simulink model "vehicle_simulation_wCOMM"  (R2018b)
settings: Solver=ode4  StartTime=0.0  StopTime=2  FixedStep=0.001  RelTol=1e-3
undefined symbols (not defined in the file): HDBK, MIL, serial
libraries: powerlib_meascontrol x7, aerolibconvert2 x5, aerolibatmos2 x3, instrumentlib x3, dspsrcs4 x2, simulink x1
(part 2 of 5)

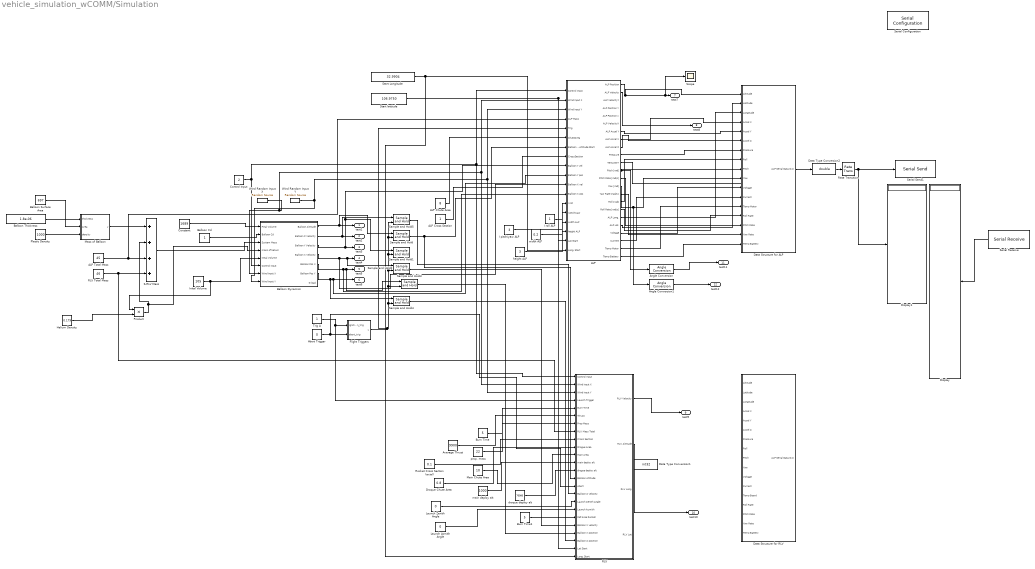
== system vehicle_simulation_wCOMM/Simulation ==
  ALP : Subsystem  TreatAsAtomicUnit=on
  ALP Chute Area : Constant  Value=8
  ALP Cross Section : Constant
  ALP Total Mass : Constant  Value=45
  Abort Trigger : Constant  Value=0
  Angle Conversion : aerolibconvert2/Angle Conversion  IU=rad  OU=deg
  Angle Conversion1 : aerolibconvert2/Angle Conversion  IU=rad  OU=deg
  Average Thrust : Constant  Value=9900
  Balloon Cd : Constant
  Balloon Dynamics : Subsystem  TreatAsAtomicUnit=on
  Balloon Surface Area : Constant  Value=697
  Balloon Thickness : Constant  Value=1.8e-06
  Burn Time : Constant  Value=5
  Burn Time1 : Constant  Value=5
  Constant : Constant  Value=1689
  Control Input : Constant  Value=2
  "Data Structure for ALP " : Subsystem  TreatAsAtomicUnit=on
  Data Structure for RLV : Subsystem  TreatAsAtomicUnit=on
  Data Type Conversion1 : DataTypeConversion  OutDataTypeStr=int32
  Data Type Conversion2 : DataTypeConversion  OutDataTypeStr=double
  Display : Display
  Display1 : Display
  Droque Chute Area : Constant  Value=0.8
  Flight Triggers : MATLAB Function  TreatAsAtomicUnit=on
  Helium Density : Constant  Value=0.179
  I pitch/yaw ALP : Constant  Value=3
  I roll ALP : Constant
  Inital Volume : Constant  Value=105
  Launch Azmith Angle : Constant  Value=0
  Launch Zenith Angle : Constant  Value=0
  Main Chute Area : Constant  Value=10
  Mass of Balloon : MATLAB Function  TreatAsAtomicUnit=on
  Plastic Density : Constant  Value=1000
  Product : Product
  RLV : Subsystem  TreatAsAtomicUnit=on
  RLV Total Mass : Constant  Value=46
  Rate Transition : RateTransition  OutPortSampleTime=1
  Rocket Cross Section (axial) : Constant  Value=0.1
  S-RLV Mass : Sum  Inputs=++++
  Sample and Hold{,1..5} (6 alike) : powerlib_meascontrol/Additional Components/Sample and Hold  ic=0  Ts=0
      settings: SourceProductName=Simscape Power Systems  SourceProductBaseCode=PS
  Scope : Scope
  Serial Configuration : instrumentlib/Serial Configuration  Priority=-200000  ComPortMenu=COM4  ComPort=COM4  ObjConstructor=serial('COM4');  BaudRate=9600  DataBits=8  Parity=none  StopBits=1  FlowControl=none  Timeout=10  ByteOrder=LittleEndian
  Serial Receive : instrumentlib/Serial Receive  ComPortMenu=COM4  ComPort=COM4  ObjConstructor=serial('COM4');  Terminator=<none>  DataSize="[1  25]"  DataType=double  EnableBlockingMode=on  ActionDataUnavailable=Output last received value  CustomValue=0  SampleTime=2
  Serial Send1 : instrumentlib/Serial Send  ComPortMenu=COM4  ComPort=COM4  ObjConstructor=serial('COM4');  Terminator=<none>  EnableBlockingMode=on
  Start Longitude : Constant  Value=32.9904
  Start lattiude : Constant  Value=106.9750
  Trig A : Constant
  Wind Random Input X : dspsrcs4/Random Source  SrcType=Gaussian  NormMethod=Ziggurat  CltLength=12  MinVal=0  MaxVal=1  MeanVal=1  VarVal=1  RepMode=Not repeatable  rawSeed=1  IsInherit=off  SampMode=Discrete  SampTime=5000  SampFrame=1  DataType=Double  OutComplex=Real  OutputFrames=off
  Wind Random Input Y : dspsrcs4/Random Source  SrcType=Gaussian  NormMethod=Ziggurat  CltLength=12  MinVal=0  MaxVal=1  MeanVal=1  VarVal=1  RepMode=Not repeatable  rawSeed=1  IsInherit=off  SampMode=Discrete  SampTime=5000  SampFrame=1  DataType=Double  OutComplex=Real  OutputFrames=off
  droque deploy alt : Constant  Value=70000
  height ALP : Constant  Value=3
  main deploy alt : Constant  Value=1000
  prop. mass : Constant  Value=22
  width ALP : Constant  Value=0.2
  test1 : Outport
  test2 : Outport  Port=2
  test3 : Outport  Port=3
  test4 : Outport  Port=4
  test5 : Outport  Port=5
  test6 : Outport  Port=6
  test7 : Outport  Port=7
  test8 : Outport  Port=8
  test9 : Outport  Port=9
  test10 : Outport  Port=10
  test11 : Outport  Port=11
  test12 : Outport  Port=12
  wires:
  Inital Volume/1 -> Product/1, Balloon Dynamics/5(Inital Volume)
  Trig A/1 -> RLV/4(Launch Trigger), Flight Triggers/1(ignition_trig)
  Balloon Dynamics/1(Balloon Altitude) -> Sample and Hold/1, test1/1
  Constant/1 -> Balloon Dynamics/1(Final Volume)
  Abort Trigger/1 -> RLV/15(Abort), Flight Triggers/2(abort_trig)
  Balloon Cd/1 -> Balloon Dynamics/2(Balloon Cd)
  RLV Total Mass/1 -> RLV/8(RLV Mass Total), S-RLV Mass/4
  ALP Total Mass/1 -> ALP/4(ALP Mass), S-RLV Mass/3
  S-RLV Mass/1 -> Balloon Dynamics/3(System Mass)
  Balloon Dynamics/2(Balloon Z Velocity) -> Sample and Hold5/1, test2/1
  Wind Random Input X/1 -> Balloon Dynamics/7(Wind Input X), RLV/2(Wind Input X), ALP/2(Wind Input X)
  Wind Random Input Y/1 -> Balloon Dynamics/8(Wind Input Y), RLV/3(Wind Input Y), ALP/3(Wind Input Y)
  Control Input/1 -> Balloon Dynamics/6(Control Input), RLV/1(Control Input), ALP/1(Control Input)
  Balloon Dynamics/3(Balloon Y Velocity) -> ALP/9(Balloon Y vel), Sample and Hold1/1, test3/1
  Balloon Dynamics/5(Balloon Pos X) -> ALP/12(Balloon X pos), Sample and Hold3/1, test5/1
  Helium Density/1 -> Product/2
  Product/1 -> Balloon Dynamics/4(mass of helium), S-RLV Mass/2
  Balloon Thickness/1 -> Mass of Balloon/1(thickness)
  Plastic Density/1 -> Mass of Balloon/3(density)
  Mass of Balloon/1(y) -> S-RLV Mass/1
  Balloon Dynamics/4(Balloon X Velocity) -> ALP/11(Balloon X vel), Sample and Hold2/1, test4/1
  Balloon Dynamics/6(Balloon Pos Y) -> Sample and Hold4/1, ALP/10(Balloon Y pos), test6/1
  Sample and Hold/1 -> RLV/14(Balloon Altitude), ALP/7(Balloon Altitude Start)
  ALP Chute Area/1 -> ALP/6(ChuteArea)
  ALP/1(ALP Position) -> "Data Structure for ALP "/1(Altitude), Scope/1, test7/1
  ALP/2(ALP Velocity) -> test8/1
  ALP Cross Section/1 -> ALP/8(CrossSection)
  Flight Triggers/1(y) -> ALP/5(Trig), Sample and Hold4/2, Sample and Hold3/2, Sample and Hold2/2, Sample and Hold1/2, Sample and Hold5/2, Sample and Hold/2
  Burn Time/1 -> RLV/5(Burn Time)
  Average Thrust/1 -> RLV/6(Thrust)
  prop. mass/1 -> RLV/7(Prop Mass)
  Rocket Cross Section (axial)/1 -> RLV/9(Cross Section)
  Droque Chute Area/1 -> RLV/10(Drogue Area)
  Main Chute Area/1 -> RLV/11(Main Area)
  main deploy alt/1 -> RLV/12(main deploy alt)
  droque deploy alt/1 -> RLV/13(drogue deploy alt)
  RLV/1(RLV Velocity) -> test9/1
  RLV/2(RLV Altitude) -> test10/1
  Balloon Surface Area/1 -> Mass of Balloon/2(Area)
  ALP/8(ALP Accel X) -> "Data Structure for ALP "/4(Accel X)
  ALP/7(ALP Accel Y) -> "Data Structure for ALP "/5(Accel Y)
  ALP/9(ALP Accel Z) -> "Data Structure for ALP "/6(Accel Z)
  I roll ALP/1 -> ALP/13(I roll)
  I pitch/yaw ALP/1 -> ALP/14(I pitch/yaw)
  width ALP/1 -> ALP/15(width ALP)
  height ALP/1 -> ALP/16(height ALP)
  ALP/14(Yaw [rad]) -> "Data Structure for ALP "/10(Yaw), Angle Conversion1/1
  ALP/12(Pitch [rad]) -> Angle Conversion/1, "Data Structure for ALP "/9(Pitch)
  Angle Conversion/1 -> test11/1
  Angle Conversion1/1 -> test12/1
  ALP/10(Pressure) -> "Data Structure for ALP "/7(Pressure)
  ALP/18(ALP Long.) -> "Data Structure for ALP "/3(Longitude)
  ALP/19(ALP Lat.) -> "Data Structure for ALP "/2(Latitude)
  ALP/16(Roll [rad]) -> "Data Structure for ALP "/8(Roll)
  ALP/13(Pitch Rate [rad/s]) -> "Data Structure for ALP "/15(Pitch Rate)
  ALP/15(Yaw Rate [rad/s]) -> "Data Structure for ALP "/16(Yaw Rate)
  ALP/17(Roll Rate [rad/s]) -> "Data Structure for ALP "/14(Roll Rate)
  ALP/11(Temp EXT) -> ?
  ALP/20(Voltage) -> "Data Structure for ALP "/11(Voltage)
  ALP/21(Current) -> "Data Structure for ALP "/12(Current)
  ALP/22(Temp Motor) -> "Data Structure for ALP "/13(Temp Motor)
  ALP/23(Temp Battery) -> "Data Structure for ALP "/17(Temp Battery)
  Start lattiude/1 -> RLV/23(Lat Start), ALP/17(Lat Start)
  Start Longitude/1 -> RLV/24(Long. Start), ALP/18(Long. Start)
  Sample and Hold3/1 -> RLV/21(Balloon X position)
  Sample and Hold4/1 -> RLV/22(Balloon Z position)
  Sample and Hold2/1 -> RLV/20(Balloon X velocity)
  Sample and Hold5/1 -> RLV/16(Balloon Z velocity)
  Burn Time1/1 -> RLV/19(Ref Area Rocket)
  Launch Zenith Angle/1 -> RLV/17(Launch Zenith Angle)
  Launch Azmith Angle/1 -> RLV/18(Launch Azmith)
  "Data Structure for ALP "/1(ALP Serial Data Out) -> Data Type Conversion2/1
  Data Type Conversion2/1 -> Rate Transition/1
  Serial Receive/1 -> Display/1
  Rate Transition/1 -> Display1/1, Serial Send1/1

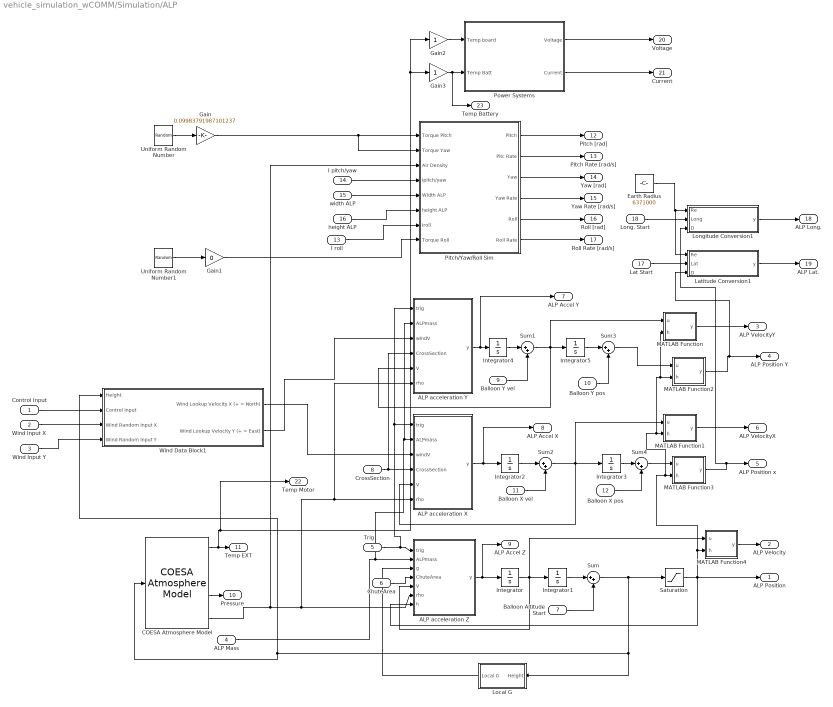
== system vehicle_simulation_wCOMM/Simulation/ALP ==
  Control Input : Inport
  Wind Input X : Inport  Port=2
  Wind Input Y : Inport  Port=3
  ALP Mass : Inport  Port=4
  Trig : Inport  Port=5
  ChuteArea : Inport  Port=6
  Balloon Altitude Start : Inport  Port=7
  CrossSection : Inport  Port=8
  Balloon Y vel : Inport  Port=9
  Balloon Y pos : Inport  Port=10
  Balloon X vel : Inport  Port=11
  Balloon X pos : Inport  Port=12
  I roll : Inport  Port=13
  I pitch/yaw : Inport  Port=14
  width ALP : Inport  Port=15
  height ALP : Inport  Port=16
  Lat Start : Inport  Port=17
  Long. Start : Inport  Port=18
  ALP acceleration X : MATLAB Function  TreatAsAtomicUnit=on
  ALP acceleration Y : MATLAB Function  TreatAsAtomicUnit=on
  ALP acceleration Z : MATLAB Function  TreatAsAtomicUnit=on
  COESA Atmosphere Model : aerolibatmos2/COESA Atmosphere Model  units=Metric (MKS)  spec=1976 COESA-extended U.S. Standard Atmosphere  model=Profile  profile_var=High temperature  profile_percent=1%  profile_alt=5 km (16404 ft)  envelope_var=High temperature  envelope_percent=1%  action=Warning
  Earth Radius : Constant  Value=6371000
  Gain : Gain  Gain=0.09983791987101237
  Gain1 : Gain  Gain=0
  Gain2 : Gain
  Gain3 : Gain
  Integrator{,1..5} (6 alike) : Integrator
  Latitude Conversion1 : MATLAB Function  TreatAsAtomicUnit=on
  Local G : Subsystem
  Longitude Conversion1 : MATLAB Function  TreatAsAtomicUnit=on
  MATLAB Function : MATLAB Function  TreatAsAtomicUnit=on
  MATLAB Function1 : MATLAB Function  TreatAsAtomicUnit=on
  MATLAB Function2 : MATLAB Function  TreatAsAtomicUnit=on
  MATLAB Function3 : MATLAB Function  TreatAsAtomicUnit=on
  MATLAB Function4 : MATLAB Function  TreatAsAtomicUnit=on
  Pitch/Yaw/Roll Sim : Subsystem  TreatAsAtomicUnit=on
  Power Systems : Subsystem  TreatAsAtomicUnit=on
  Saturation : Saturate  UpperLimit=inf  LowerLimit=0
  Sum{,1..4} (5 alike) : Sum  Inputs=|++
  Uniform Random Number : UniformRandomNumber  SampleTime=0.2
  Uniform Random Number1 : UniformRandomNumber  SampleTime=0.3
  Wind Data Block1 : Subsystem
  ALP Position : Outport
  ALP Velocity : Outport  Port=2
  ALP VelocityY : Outport  Port=3
  ALP Position Y : Outport  Port=4
  ALP Position x : Outport  Port=5
  ALP VelocityX : Outport  Port=6
  ALP Accel Y : Outport  Port=7
  ALP Accel X : Outport  Port=8
  ALP Accel Z : Outport  Port=9
  Pressure : Outport  Port=10
  Temp EXT : Outport  Port=11
  Pitch [rad] : Outport  Port=12
  Pitch Rate [rad/s] : Outport  Port=13
  Yaw [rad] : Outport  Port=14
  Yaw Rate [rad/s] : Outport  Port=15
  Roll [rad] : Outport  Port=16
  Roll Rate [rad/s] : Outport  Port=17
  ALP Long. : Outport  Port=18
  ALP Lat. : Outport  Port=19
  Voltage : Outport  Port=20
  Current : Outport  Port=21
  Temp Motor : Outport  Port=22
  Temp Battery : Outport  Port=23
  wires:
  Wind Input Y/1 -> Wind Data Block1/4(Wind Random Input Y)
  Control Input/1 -> Wind Data Block1/2(Control Input)
  Wind Input X/1 -> Wind Data Block1/3(Wind Random Input X)
  ALP acceleration Z/1(y) -> ALP Accel Z/1, Integrator/1
  Integrator/1 -> MATLAB Function4/1(u), ALP acceleration Z/5(V), Integrator1/1
  Local G/1(Local G) -> ALP acceleration Z/3(g)
  ALP Mass/1 -> ALP acceleration Y/2(ALPmass), ALP acceleration X/2(ALPmass), ALP acceleration Z/2(ALPmass)
  Trig/1 -> ALP acceleration Y/1(trig), ALP acceleration X/1(trig), ALP acceleration Z/1(trig)
  COESA Atmosphere Model/4 -> Pitch/Yaw/Roll Sim/3(Air Density), ALP acceleration Y/6(rho), ALP acceleration X/6(rho), ALP acceleration Z/6(rho)
  ChuteArea/1 -> ALP acceleration Z/4(ChuteArea)
  Integrator1/1 -> Sum/1
  Sum/1 -> Wind Data Block1/1(Height), COESA Atmosphere Model/1, Local G/1(Height), Saturation/1
  Balloon Altitude Start/1 -> Sum/2
  CrossSection/1 -> ALP acceleration Y/4(CrossSection), ALP acceleration X/4(CrossSection)
  Wind Data Block1/1(Wind Lookup Velocity X (+ = North)) -> ALP acceleration X/3(windV)
  ALP acceleration X/1(y) -> ALP Accel X/1, Integrator2/1
  Wind Data Block1/2(Wind Lookup Velocity Y (+ = East)) -> ALP acceleration Y/3(windV)
  ALP acceleration Y/1(y) -> ALP Accel Y/1, Integrator4/1
  Integrator4/1 -> Sum1/1
  Sum1/1 -> MATLAB Function/1(u), ALP acceleration Y/5(V), Integrator5/1
  Integrator2/1 -> Sum2/1
  Sum2/1 -> MATLAB Function1/1(u), ALP acceleration X/5(V), Integrator3/1
  Integrator5/1 -> Sum3/1
  Integrator3/1 -> Sum4/1
  Balloon Y vel/1 -> Sum1/2
  Balloon Y pos/1 -> Sum3/2
  Balloon X vel/1 -> Sum2/2
  Balloon X pos/1 -> Sum4/2
  MATLAB Function/1(y) -> ALP VelocityY/1
  MATLAB Function2/1(y) -> Latitude Conversion1/3(D), ALP Position Y/1
  Saturation/1 -> MATLAB Function/2(h), MATLAB Function2/2(h), MATLAB Function1/2(h), MATLAB Function3/2(h), MATLAB Function4/2(h), ALP acceleration Z/7(h), ALP Position/1
  MATLAB Function1/1(y) -> ALP VelocityX/1
  MATLAB Function3/1(y) -> ALP Position x/1, Longitude Conversion1/3(D)
  MATLAB Function4/1(y) -> ALP Velocity/1
  Sum3/1 -> MATLAB Function2/1(u)
  Sum4/1 -> MATLAB Function3/1(u)
  COESA Atmosphere Model/3 -> Pressure/1
  COESA Atmosphere Model/1 -> Temp Motor/1, Gain3/1, Gain2/1, Temp EXT/1
  I roll/1 -> Pitch/Yaw/Roll Sim/7(Iroll)
  I pitch/yaw/1 -> Pitch/Yaw/Roll Sim/4(Ipitch/yaw)
  width ALP/1 -> Pitch/Yaw/Roll Sim/5(Width ALP)
  height ALP/1 -> Pitch/Yaw/Roll Sim/6(height ALP)
  Pitch/Yaw/Roll Sim/1(Pitch) -> Pitch [rad]/1
  Pitch/Yaw/Roll Sim/2(Pitc Rate) -> Pitch Rate [rad/s]/1
  Pitch/Yaw/Roll Sim/3(Yaw) -> Yaw [rad]/1
  Pitch/Yaw/Roll Sim/4(Yaw Rate) -> Yaw Rate [rad/s]/1
  Pitch/Yaw/Roll Sim/5(Roll) -> Roll [rad]/1
  Pitch/Yaw/Roll Sim/6(Roll Rate) -> Roll Rate [rad/s]/1
  Uniform Random Number/1 -> Gain/1
  Gain/1 -> Pitch/Yaw/Roll Sim/2(Torque Yaw), Pitch/Yaw/Roll Sim/1(Torque Pitch)
  Uniform Random Number1/1 -> Gain1/1
  Gain1/1 -> Pitch/Yaw/Roll Sim/8(Torque Roll)
  Lat Start/1 -> Latitude Conversion1/2(Lat)
  Long. Start/1 -> Longitude Conversion1/2(Long)
  Earth Radius/1 -> Latitude Conversion1/1(Re), Longitude Conversion1/1(Re)
  Longitude Conversion1/1(y) -> ALP Long./1
  Latitude Conversion1/1(y) -> ALP Lat./1
  Power Systems/1(Voltage) -> Voltage/1
  Power Systems/2(Current) -> Current/1
  Gain2/1 -> Power Systems/1(Temp board)
  Gain3/1 -> Temp Battery/1, Power Systems/2(Temp Batt)

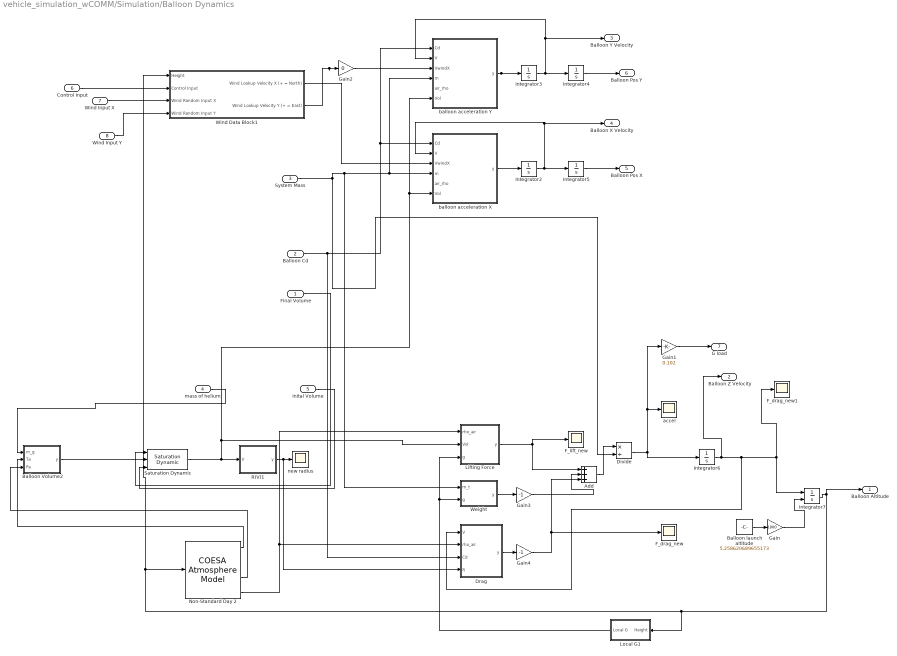
== system vehicle_simulation_wCOMM/Simulation/Balloon Dynamics ==
  Final Volume : Inport
  Balloon Cd : Inport  Port=2
  System Mass : Inport  Port=3
  mass of helium : Inport  Port=4
  Inital Volume : Inport  Port=5
  Control Input : Inport  Port=6
  Wind Input X : Inport  Port=7
  Wind Input Y : Inport  Port=8
  Add : Sum  Inputs=+++
  Balloon Volume2 : MATLAB Function  TreatAsAtomicUnit=on
  Balloon launch altitude : Constant  Value=5.258620689655173
  Divide : Product  Inputs=*/
  Drag : MATLAB Function  TreatAsAtomicUnit=on
  F_drag_new : Scope
  F_drag_new1 : Scope
  F_lift_new : Scope
  Gain : Gain  Gain=1000
  Gain1 : Gain  Gain=0.102
  Gain2 : Gain  Gain=0
  Gain3 : Gain  Gain=-1
  Gain4 : Gain  Gain=-1
  Integrator{2..6} (5 alike) : Integrator
  Integrator7 : Integrator  InitialConditionSource=external
  Lifting Force : MATLAB Function  TreatAsAtomicUnit=on
  Local G1 : Subsystem
  Non-Standard Day 2 : aerolibatmos2/COESA Atmosphere Model  units=Metric (MKS)  spec=MIL-HDBK-310  model=Profile  profile_var=High temperature  profile_percent=1%  profile_alt=5 km (16404 ft)  envelope_var=High temperature  envelope_percent=1%  action=Warning
  R(V)1 : MATLAB Function  TreatAsAtomicUnit=on
  Saturation Dynamic : simulink/Discontinuities/Saturation Dynamic  OutMin=[]  OutMax=[]  OutDataTypeStr=Inherit: Same as second input  OutDataType=fixdt(1, 16)  OutScaling=2^-10  DoSatur=off
  Weight : MATLAB Function  TreatAsAtomicUnit=on
  Wind Data Block1 : Subsystem
  accel : Scope
  balloon acceleration X : MATLAB Function  TreatAsAtomicUnit=on
  balloon acceleration Y : MATLAB Function  TreatAsAtomicUnit=on
  new radius : Scope
  Balloon Altitude : Outport
  Balloon Z Velocity : Outport  Port=2
  Balloon Y Velocity : Outport  Port=3
  Balloon X Velocity : Outport  Port=4
  Balloon Pos X : Outport  Port=5
  Balloon Pos Y : Outport  Port=6
  G load : Outport  Port=7
  wires:
  Balloon Cd/1 -> Drag/3(Cd), balloon acceleration Y/1(Cd), balloon acceleration X/1(Cd)
  mass of helium/1 -> Balloon Volume2/1(m_g)
  Balloon Volume2/1(y) -> Saturation Dynamic/2
  Final Volume/1 -> Saturation Dynamic/1
  Inital Volume/1 -> Saturation Dynamic/3
  balloon acceleration X/1(y) -> Integrator2/1
  balloon acceleration Y/1(y) -> Integrator3/1
  Integrator3/1 -> Balloon Y Velocity/1, balloon acceleration Y/2(V), Integrator4/1
  Integrator2/1 -> Balloon X Velocity/1, balloon acceleration X/2(V), Integrator5/1
  Integrator5/1 -> Balloon Pos X/1
  Integrator4/1 -> Balloon Pos Y/1
  Wind Data Block1/2(Wind Lookup Velocity Y (+ = East)) -> Gain2/1
  Wind Data Block1/1(Wind Lookup Velocity X (+ = North)) -> balloon acceleration X/3(VwindX)
  Control Input/1 -> Wind Data Block1/2(Control Input)
  Wind Input X/1 -> Wind Data Block1/3(Wind Random Input X)
  Wind Input Y/1 -> Wind Data Block1/4(Wind Random Input Y)
  System Mass/1 -> Weight/1(m_t), balloon acceleration Y/4(m), balloon acceleration X/4(m), Divide/2
  Saturation Dynamic/1 -> R(V)1/1(V), Lifting Force/2(Vol), balloon acceleration Y/6(Vol), balloon acceleration X/6(Vol)
  Gain3/1 -> Add/2
  Add/1 -> Divide/1
  Divide/1 -> Gain1/1, accel/1, Integrator6/1
  R(V)1/1(y) -> Drag/4(R), new radius/1
  Gain2/1 -> balloon acceleration Y/3(VwindX)
  Drag/1(y) -> Gain4/1
  Weight/1(y) -> Gain3/1
  Gain4/1 -> Add/3, F_drag_new/1
  Lifting Force/1(y) -> Add/1, F_lift_new/1
  Integrator7/1 -> Local G1/1(Height), Wind Data Block1/1(Height), Non-Standard Day 2/1, Balloon Altitude/1
  Non-Standard Day 2/3 -> Balloon Volume2/3(Pa)
  Non-Standard Day 2/1 -> Balloon Volume2/2(Ta)
  Non-Standard Day 2/4 -> Drag/2(rho_air), Lifting Force/1(rho_air)
  Local G1/1(Local G) -> Lifting Force/3(g), Weight/2(g)
  Integrator6/1 -> Drag/1(V), F_drag_new1/1, Integrator7/1, Balloon Z Velocity/1
  Balloon launch altitude/1 -> Gain/1
  Gain/1 -> Integrator7/2
  Gain1/1 -> G load/1

== system vehicle_simulation_wCOMM/Simulation/Data Structure for ALP  ==
  Altitude : Inport
  Latitude : Inport  Port=2
  Longitude : Inport  Port=3
  Accel X : Inport  Port=4
  Accel Y : Inport  Port=5
  Accel Z : Inport  Port=6
  Pressure : Inport  Port=7
  Roll : Inport  Port=8
  Pitch : Inport  Port=9
  Yaw : Inport  Port=10
  Voltage : Inport  Port=11
  Current : Inport  Port=12
  Temp Motor : Inport  Port=13
  Roll Rate : Inport  Port=14
  Pitch Rate : Inport  Port=15
  Yaw Rate : Inport  Port=16
  Temp Battery : Inport  Port=17
  Abs{2..5} (4 alike) : Abs
  Display1 : Display
  Gain{,1..5} (6 alike) : Gain  Gain=10000
  Vector Concatenate : Concatenate  NumInputs=17
  ALP Serial Data Out : Outport
  wires:
  Altitude/1 -> Vector Concatenate/1
  Vector Concatenate/1 -> ALP Serial Data Out/1, Display1/1
  Latitude/1 -> Vector Concatenate/2
  Longitude/1 -> Vector Concatenate/3
  Accel X/1 -> Vector Concatenate/4
  Accel Y/1 -> Vector Concatenate/5
  Accel Z/1 -> Vector Concatenate/6
  Roll/1 -> Abs2/1
  Pitch/1 -> Gain/1
  Abs2/1 -> Gain2/1
  Gain/1 -> Vector Concatenate/7
  Gain1/1 -> Vector Concatenate/8
  Yaw/1 -> Gain1/1
  Roll Rate/1 -> Abs3/1
  Pitch Rate/1 -> Abs4/1
  Yaw Rate/1 -> Abs5/1
  Abs3/1 -> Gain3/1
  Abs4/1 -> Gain4/1
  Abs5/1 -> Gain5/1
  Gain2/1 -> Vector Concatenate/9
  Gain3/1 -> Vector Concatenate/10
  Gain4/1 -> Vector Concatenate/11
  Gain5/1 -> Vector Concatenate/12
  Pressure/1 -> Vector Concatenate/13
  Temp Motor/1 -> Vector Concatenate/14
  Temp Battery/1 -> Vector Concatenate/15
  Voltage/1 -> Vector Concatenate/16
  Current/1 -> Vector Concatenate/17

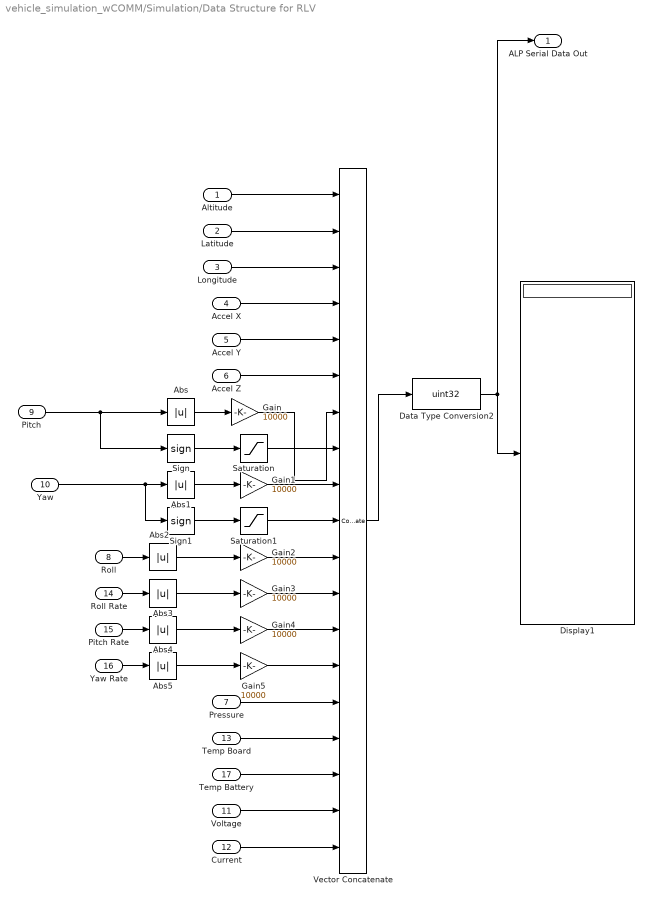
== system vehicle_simulation_wCOMM/Simulation/Data Structure for RLV ==
  Altitude : Inport
  Latitude : Inport  Port=2
  Longitude : Inport  Port=3
  Accel X : Inport  Port=4
  Accel Y : Inport  Port=5
  Accel Z : Inport  Port=6
  Pressure : Inport  Port=7
  Roll : Inport  Port=8
  Pitch : Inport  Port=9
  Yaw : Inport  Port=10
  Voltage : Inport  Port=11
  Current : Inport  Port=12
  Temp Board : Inport  Port=13
  Roll Rate : Inport  Port=14
  Pitch Rate : Inport  Port=15
  Yaw Rate : Inport  Port=16
  Temp Battery : Inport  Port=17
  Abs{,1..5} (6 alike) : Abs
  Data Type Conversion2 : DataTypeConversion  OutDataTypeStr=uint32
  Display1 : Display
  Gain{,1..5} (6 alike) : Gain  Gain=10000
  Saturation : Saturate  UpperLimit=1  LowerLimit=0
  Saturation1 : Saturate  UpperLimit=1  LowerLimit=0
  Sign : Signum
  Sign1 : Signum
  Vector Concatenate : Concatenate  NumInputs=19
  ALP Serial Data Out : Outport
  wires:
  Altitude/1 -> Vector Concatenate/1
  Vector Concatenate/1 -> Data Type Conversion2/1
  Data Type Conversion2/1 -> ALP Serial Data Out/1, Display1/1
  Latitude/1 -> Vector Concatenate/2
  Longitude/1 -> Vector Concatenate/3
  Accel X/1 -> Vector Concatenate/4
  Accel Y/1 -> Vector Concatenate/5
  Accel Z/1 -> Vector Concatenate/6
  Pitch/1 -> Abs/1, Sign/1
  Yaw/1 -> Abs1/1, Sign1/1
  Roll/1 -> Abs2/1
  Abs/1 -> Gain/1
  Sign1/1 -> Saturation1/1
  Abs1/1 -> Gain1/1
  Abs2/1 -> Gain2/1
  Gain/1 -> Vector Concatenate/7
  Gain1/1 -> Vector Concatenate/9
  Sign/1 -> Saturation/1
  Saturation/1 -> Vector Concatenate/8
  Saturation1/1 -> Vector Concatenate/10
  Roll Rate/1 -> Abs3/1
  Pitch Rate/1 -> Abs4/1
  Yaw Rate/1 -> Abs5/1
  Abs3/1 -> Gain3/1
  Abs4/1 -> Gain4/1
  Abs5/1 -> Gain5/1
  Pressure/1 -> Vector Concatenate/15
  Temp Board/1 -> Vector Concatenate/16
  Temp Battery/1 -> Vector Concatenate/17
  Voltage/1 -> Vector Concatenate/18
  Current/1 -> Vector Concatenate/19
  Gain2/1 -> Vector Concatenate/11
  Gain3/1 -> Vector Concatenate/12
  Gain4/1 -> Vector Concatenate/13
  Gain5/1 -> Vector Concatenate/14

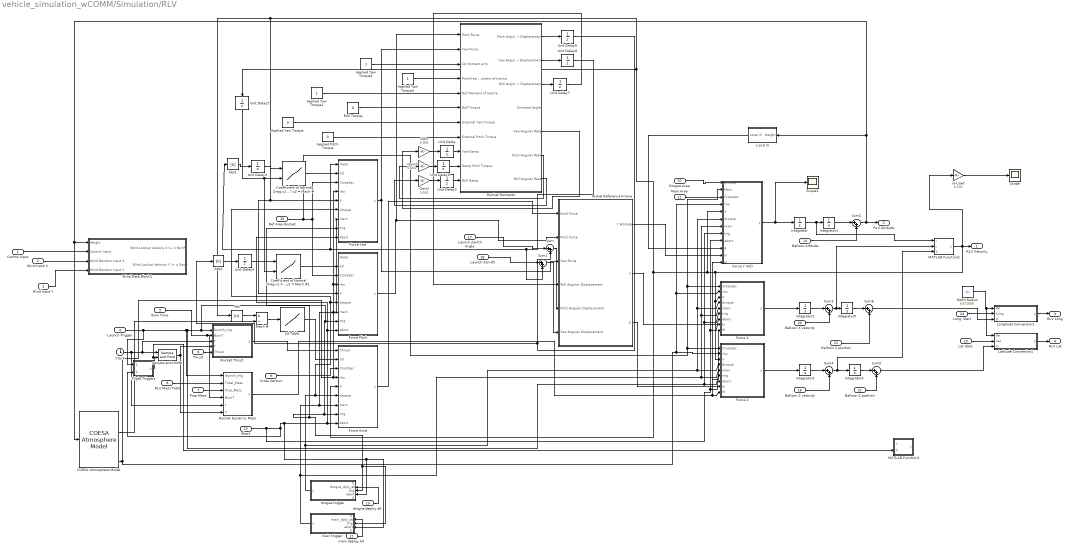
== system vehicle_simulation_wCOMM/Simulation/RLV ==
  Control Input : Inport
  Wind Input X : Inport  Port=2
  Wind Input Y : Inport  Port=3
  Launch Trigger : Inport  Port=4
  Burn Time : Inport  Port=5
  Thrust : Inport  Port=6
  Prop Mass : Inport  Port=7
  RLV Mass Total : Inport  Port=8
  Cross Section : Inport  Port=9
  Drogue Area : Inport  Port=10
  Main Area : Inport  Port=11
  main deploy alt : Inport  Port=12
  drogue deploy alt : Inport  Port=13
  Balloon Altitude : Inport  Port=14
  Abort : Inport  Port=15
  Balloon Z velocity : Inport  Port=16
  Launch Zenith Angle : Inport  Port=17
  Launch Azmith : Inport  Port=18
  Ref Area Rocket : Inport  Port=19
  Balloon X velocity : Inport  Port=20
  Balloon X position : Inport  Port=21
  Balloon Z position : Inport  Port=22
  Lat Start : Inport  Port=23
  Long. Start : Inport  Port=24
  Abs : Abs
  Abs1 : Abs
  Abs2 : Abs
  Applied Pitch Torque : Constant  Value=0
  Applied Yaw Torque : Constant  Value=0
  Applied Yaw Torque1 : Constant
  Applied Yaw Torque2 : Constant
  Applied Yaw Torque3 : Constant
  COESA Atmosphere Model : aerolibatmos2/COESA Atmosphere Model  units=Metric (MKS)  spec=1976 COESA-extended U.S. Standard Atmosphere  model=Profile  profile_var=High temperature  profile_percent=1%  profile_alt=5 km (16404 ft)  envelope_var=High temperature  envelope_percent=1%  action=Warning
  Cd Table : Lookup_n-D  NumberOfTableDimensions=1  BreakpointsForDimension1=[0,0.05,0.1,0.6,0.9,1.1,1.2,2,3,4,5]  Table=[0.48,0.4,0.42,0.4,0.44,0.54,0.52,0.36,0.24,0.18,0.14]  InternalRulePriority=Speed  RndMeth=Simplest  InputSameDT=on
  Clock : Clock
  Coefficient of Normal Drag u1 = AOA (Degrees) u2 = Mach # : Lookup_n-D  BreakpointsForDimension1=[0,2,4,6,8,10,12,14,15]  BreakpointsForDimension2=[0,0.5,1.1,2,5]  Table=reshape([1e-06,0.6,1.25,1.9,2.5,3.2,3.6,4.2,4.5,1e-06,0.6,1.25,1.9,2.5,3.2,3.6,4.2,4.5,1e-06,0.8,1.6,2.5,3.4,4.2,5,5.8,6.2,1e-06,0.7,1.4,2,2.5,3.2,4,5.6,6.2,1e-06,0.25,0.8,1.4,2,2.6,3.2,3.9,3.3],9,5)  UseLastTableValue=on  InternalRulePriority=Speed  RndMeth=Simplest  InputSameDT=on
  Coefficient of Normal Drag u1 = AOA (Degrees) u2 = Mach #1 : Lookup_n-D  BreakpointsForDimension1=[0,2,4,6,8,10,12,14,15]  BreakpointsForDimension2=[0,0.5,1.1,2,5]  Table=reshape([1e-06,0.6,1.25,1.9,2.5,3.2,3.6,4.2,4.5,1e-06,0.6,1.25,1.9,2.5,3.2,3.6,4.2,4.5,1e-06,0.8,1.6,2.5,3.4,4.2,5,5.8,6.2,1e-06,0.7,1.4,2,2.5,3.2,4,5.6,6.2,1e-06,0.25,0.8,1.4,2,2.6,3.2,3.9,3.3],9,5)  UseLastTableValue=on  InternalRulePriority=Speed  RndMeth=Simplest  InputSameDT=on
  Earth Radius : Constant  Value=6371000
  Flight Triggers : MATLAB Function  TreatAsAtomicUnit=on
  Force Axial : MATLAB Function  TreatAsAtomicUnit=on
  Force Pitch : MATLAB Function  TreatAsAtomicUnit=on
  Force X : MATLAB Function  TreatAsAtomicUnit=on
  Force Y (alt) : MATLAB Function  TreatAsAtomicUnit=on
  Force Yaw : MATLAB Function  TreatAsAtomicUnit=on
  Force Z : MATLAB Function  TreatAsAtomicUnit=on
  G-Load : Gain  Gain=0.101
  Gain : Gain  Gain=0.001
  Gain2 : Gain  Gain=0.001
  Gain3 : Gain  Gain=0.001
  Global Reference Frame : Subsystem  TreatAsAtomicUnit=on
  Integrator{,1..5} (6 alike) : Integrator
  Latitude Conversion1 : MATLAB Function  TreatAsAtomicUnit=on
  Local G : Subsystem
  Longitude Conversion1 : MATLAB Function  TreatAsAtomicUnit=on
  MATLAB Function1 : MATLAB Function  TreatAsAtomicUnit=on
  MATLAB Function2 : MATLAB Function  TreatAsAtomicUnit=on
  Mach # : Product  Inputs=*/
  Rocket Dynamic Mass : MATLAB Function  TreatAsAtomicUnit=on
  Rocket Moments : Subsystem  TreatAsAtomicUnit=on
  Rocket Thrust : MATLAB Function  TreatAsAtomicUnit=on
  Roll Torque : Constant  Value=0
  Sample and Hold6 : powerlib_meascontrol/Additional Components/Sample and Hold  ic=0  Ts=0
      settings: SourceProductName=Simscape Power Systems  SourceProductBaseCode=PS
  Scope : Scope
  Scope1 : Scope
  Sum{,1..6} (7 alike) : Sum  Inputs=|++
  Unit Delay{,1..8} (9 alike) : UnitDelay  SampleTime=-1
  Wind Data Block1 : Subsystem
  drogue trigger : MATLAB Function  TreatAsAtomicUnit=on
  main trigger : MATLAB Function  TreatAsAtomicUnit=on
  RLV Velocity : Outport
  RLV Altitude : Outport  Port=2
  RLV Long : Outport  Port=3
  RLV Lat : Outport  Port=4
  wires:
  Wind Input Y/1 -> Wind Data Block1/4(Wind Random Input Y)
  Control Input/1 -> Wind Data Block1/2(Control Input)
  Wind Input X/1 -> Wind Data Block1/3(Wind Random Input X)
  Clock/1 -> Rocket Dynamic Mass/5(t), Sample and Hold6/1, Rocket Thrust/3(t)
  Sample and Hold6/1 -> Rocket Thrust/4(T), Rocket Dynamic Mass/6(T)
  Burn Time/1 -> Rocket Dynamic Mass/4(BurnT), Rocket Thrust/2(BurnT)
  Thrust/1 -> Rocket Thrust/5(Thrust)
  Prop Mass/1 -> Rocket Dynamic Mass/3(Prop_Mass)
  RLV Mass Total/1 -> Rocket Dynamic Mass/2(Total_Mass)
  Rocket Thrust/1(y) -> Force Axial/1(Thrust)
  COESA Atmosphere Model/4 -> Force Yaw/4(rho), Force Pitch/4(rho), Force Axial/4(rho), Force Y (alt)/4(rho), Force X/2(rho), Force Z/2(rho)
  Cross Section/1 -> Force Axial/3(CrossSec)
  Drogue Area/1 -> Force Y (alt)/1(Droque)
  Main Area/1 -> Force Y (alt)/2(Main)
  drogue trigger/1(y) -> Force X/4(droque), Force Y (alt)/6(droque), Force Z/4(droque), Force Yaw/6(droque), Force Pitch/6(droque), Force Axial/6(droque)
  main trigger/1(y) -> Force Y (alt)/7(main), Force X/5(main), Force Z/5(main), Force Yaw/7(main), Force Pitch/7(main), Force Axial/7(main)
  main deploy alt/1 -> main trigger/2(main_dply_alt)
  drogue deploy alt/1 -> drogue trigger/2(drogue_dply_alt)
  COESA Atmosphere Model/2 -> Mach #/2
  Mach #/1 -> Cd Table/1
  Cd Table/1 -> Force Axial/2(Cd)
  Flight Triggers/1(y) -> MATLAB Function1/2(h), Sample and Hold6/2
  Abs/1 -> Mach #/1
  Force Pitch/1(y) -> Rocket Moments/1(Pitch Force), Global Reference Frame/2(Pitch Force)
  Force Yaw/1(y) -> Rocket Moments/2(Yaw Force), Global Reference Frame/3(Yaw Force)
  Rocket Moments/1(Pitch Angular Displacement) -> Unit Delay6/1
  Rocket Moments/2(Yaw Angular Displacement) -> Unit Delay8/1
  Rocket Moments/3(Roll Angular Displacement) -> Unit Delay7/1
  Coefficient of Normal Drag u1 = AOA (Degrees) u2 = Mach #/1 -> Force Yaw/2(Cd)
  Abs1/1 -> Unit Delay3/1
  Coefficient of Normal Drag u1 = AOA (Degrees) u2 = Mach #1/1 -> Force Pitch/2(Cd)
  Abs2/1 -> Unit Delay4/1
  Gain/1 -> Unit Delay/1
  Gain2/1 -> Unit Delay2/1
  Gain3/1 -> Unit Delay1/1
  Rocket Moments/6(Pitch Angular Rate) -> Gain3/1
  Rocket Moments/7(Roll Angular Rate) -> Gain2/1
  Balloon Altitude/1 -> Sum2/2
  Force Axial/1(y) -> Global Reference Frame/1(Axial Force)
  Applied Yaw Torque/1 -> Rocket Moments/7(External Yaw Torque)
  Applied Pitch Torque/1 -> Rocket Moments/8(External Pitch Torque)
  Applied Yaw Torque1/1 -> Rocket Moments/5(Roll Moment of Inertia)
  Applied Yaw Torque2/1 -> Rocket Moments/4(Pitch/Yaw Moment of Inertia)
  Applied Yaw Torque3/1 -> Rocket Moments/3(Cp moment arm)
  Roll Torque/1 -> Rocket Moments/6(Roll Torque)
  Abort/1 -> Force X/7(abort), Force Y (alt)/9(abort), Force Z/7(abort), main trigger/4(abort), drogue trigger/4(abort), Force Yaw/9(abort), Force Pitch/9(abort), Force Axial/9(abort), Flight Triggers/2(abort_trig)
  Ref Area Rocket/1 -> Force Z/1(CrossSec), Force Y (alt)/3(CrossSec), Force X/1(CrossSec), Force Yaw/3(CrossSec), Force Pitch/3(CrossSec)
  Balloon Z velocity/1 -> Sum4/2
  Balloon X velocity/1 -> Sum3/2
  Balloon Z position/1 -> Sum5/2
  Balloon X position/1 -> Sum6/2
  Launch Zenith Angle/1 -> Sum/1
  Launch Azmith/1 -> Sum1/1
  Sum/1 -> Global Reference Frame/5(Pitch Angular Displacement)
  Sum1/1 -> Global Reference Frame/6(Yaw Angular Displacement)
  Rocket Dynamic Mass/1(y) -> Force Y (alt)/12(M), Force Z/9(M), Force X/9(M)
  Force Y (alt)/1(y) -> Scope1/1, Integrator/1
  Local G/1(Local G) -> Force Y (alt)/10(g)
  Launch Trigger/1 -> Flight Triggers/1(ignition_trig), Force Y (alt)/8(trig), Force X/6(trig), Force Z/6(trig), main trigger/3(trig), drogue trigger/3(trig), Force Yaw/8(trig), Force Pitch/8(trig), Force Axial/8(trig), Rocket Thrust/1(launch_trig), Rocket Dynamic Mass/1(launch_trig)
  Integrator1/1 -> Sum2/1
  Integrator/1 -> MATLAB Function2/1(i), Integrator1/1
  Force X/1(y) -> Integrator2/1
  Force Z/1(y) -> Integrator3/1
  Integrator2/1 -> Sum3/1
  Integrator3/1 -> Sum4/1
  Sum4/1 -> MATLAB Function2/3(k), Integrator4/1
  Integrator4/1 -> Sum5/1
  Sum3/1 -> MATLAB Function2/2(j), Integrator5/1
  Integrator5/1 -> Sum6/1
  Earth Radius/1 -> Latitude Conversion1/1(Re), Longitude Conversion1/1(Re)
  Long. Start/1 -> Longitude Conversion1/2(Long)
  Lat Start/1 -> Latitude Conversion1/2(Lat)
  Sum6/1 -> Longitude Conversion1/3(D)
  Sum5/1 -> Latitude Conversion1/3(D)
  Sum2/1 -> Local G/1(Height), Wind Data Block1/1(Height), COESA Atmosphere Model/1, RLV Altitude/1
  Global Reference Frame/1(Y Altitude) -> Force Y (alt)/11(In)
  Global Reference Frame/2(X) -> Force X/8(In)
  Global Reference Frame/3(Z) -> Force Z/8(In)
  G-Load/1 -> Scope/1
  MATLAB Function2/1(y) -> G-Load/1, Abs/1, Force Pitch/5(V), Force Yaw/5(V), Unit Delay5/1, Force Axial/5(V), Force Y (alt)/5(V), Force Z/3(V), Force X/3(V), RLV Velocity/1
  Longitude Conversion1/1(y) -> RLV Long/1
  Latitude Conversion1/1(y) -> RLV Lat/1
  Unit Delay/1 -> Rocket Moments/9(Yaw Damp)
  Unit Delay1/1 -> Rocket Moments/10(Damp Pitch Torque)
  Unit Delay2/1 -> Rocket Moments/11(Roll Damp)
  Unit Delay3/1 -> Coefficient of Normal Drag u1 = AOA (Degrees) u2 = Mach #/1
  Unit Delay4/1 -> Coefficient of Normal Drag u1 = AOA (Degrees) u2 = Mach #1/1
  Unit Delay5/1 -> Coefficient of Normal Drag u1 = AOA (Degrees) u2 = Mach #1/2, Coefficient of Normal Drag u1 = AOA (Degrees) u2 = Mach #/2
  Rocket Moments/5(Yaw Angular Rate) -> Gain/1
  Unit Delay7/1 -> Global Reference Frame/4(Roll Angular Displacement)
  Unit Delay8/1 -> Force Yaw/1(theta), Abs1/1, Sum1/2
  Unit Delay6/1 -> Sum/2, Abs2/1

== system vehicle_simulation_wCOMM/Simulation/ALP/Local G ==
  Height : Inport
  Add : Sum
  Air Density Approx. : Math  Operator=square  OutMin=0  OutMax=10000  SaturateOnIntegerOverflow=on
  Divide : Product  Inputs=*/
  G : Constant  Value=9.81
  Product : Product
  Radius of Earth : Constant  Value=6371000
  Local G : Outport
  wires:
  Radius of Earth/1 -> Divide/1, Add/1
  Height/1 -> Add/2
  Add/1 -> Divide/2
  Divide/1 -> Air Density Approx./1
  Air Density Approx./1 -> Product/2
  Product/1 -> Local G/1
  G/1 -> Product/1

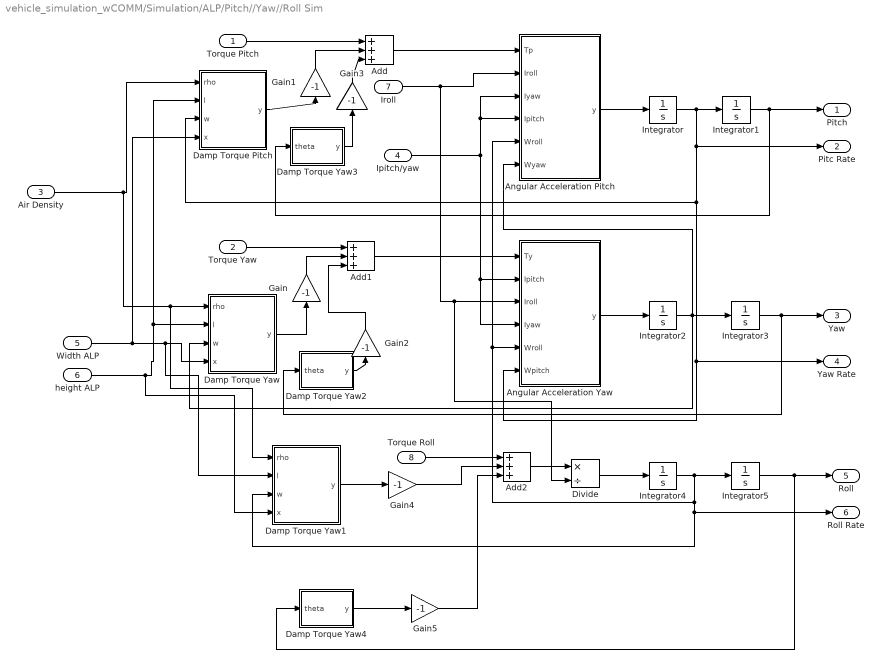
== system vehicle_simulation_wCOMM/Simulation/ALP/Pitch//Yaw//Roll Sim ==
  Torque Pitch : Inport
  Torque Yaw : Inport  Port=2
  Air Density : Inport  Port=3
  Ipitch/yaw : Inport  Port=4
  Width ALP : Inport  Port=5
  height ALP : Inport  Port=6
  Iroll : Inport  Port=7
  Torque Roll : Inport  Port=8
  Add : Sum  Inputs=+++
  Add1 : Sum  Inputs=+++
  Add2 : Sum  Inputs=+++
  Angular Acceleration Pitch : MATLAB Function  TreatAsAtomicUnit=on
  Angular Acceleration Yaw : MATLAB Function  TreatAsAtomicUnit=on
  Damp Torque Pitch : MATLAB Function  TreatAsAtomicUnit=on
  Damp Torque Yaw : MATLAB Function  TreatAsAtomicUnit=on
  Damp Torque Yaw1 : MATLAB Function  TreatAsAtomicUnit=on
  Damp Torque Yaw2 : MATLAB Function  TreatAsAtomicUnit=on
  Damp Torque Yaw3 : MATLAB Function  TreatAsAtomicUnit=on
  Damp Torque Yaw4 : MATLAB Function  TreatAsAtomicUnit=on
  Divide : Product  Inputs=*/
  Gain{,1..5} (6 alike) : Gain  Gain=-1
  Integrator{,1..5} (6 alike) : Integrator
  Pitch : Outport
  Pitc Rate : Outport  Port=2
  Yaw : Outport  Port=3
  Yaw Rate : Outport  Port=4
  Roll : Outport  Port=5
  Roll Rate : Outport  Port=6
  wires:
  Add/1 -> Angular Acceleration Pitch/1(Tp)
  Torque Pitch/1 -> Add/1
  Add1/1 -> Angular Acceleration Yaw/1(Ty)
  Torque Yaw/1 -> Add1/1
  Damp Torque Pitch/1(y) -> Gain1/1
  Damp Torque Yaw/1(y) -> Gain/1
  Air Density/1 -> Damp Torque Yaw1/1(rho), Damp Torque Yaw/1(rho), Damp Torque Pitch/1(rho)
  Ipitch/yaw/1 -> Angular Acceleration Pitch/3(Iyaw), Angular Acceleration Pitch/4(Ipitch), Angular Acceleration Yaw/4(Iyaw), Angular Acceleration Yaw/2(Ipitch)
  height ALP/1 -> Damp Torque Yaw1/4(x), Damp Torque Yaw/2(l), Damp Torque Pitch/2(l)
  Width ALP/1 -> Damp Torque Pitch/4(x), Damp Torque Yaw1/2(l), Damp Torque Yaw/4(x)
  Iroll/1 -> Divide/2, Angular Acceleration Yaw/3(Iroll), Angular Acceleration Pitch/2(Iroll)
  Gain/1 -> Add1/2
  Gain1/1 -> Add/2
  Angular Acceleration Pitch/1(y) -> Integrator/1
  Angular Acceleration Yaw/1(y) -> Integrator2/1
  Integrator2/1 -> Damp Torque Yaw/3(w), Angular Acceleration Pitch/6(Wyaw), Integrator3/1
  Torque Roll/1 -> Add2/1
  Damp Torque Yaw1/1(y) -> Gain4/1
  Add2/1 -> Divide/1
  Divide/1 -> Integrator4/1
  Integrator4/1 -> Angular Acceleration Pitch/5(Wroll), Angular Acceleration Yaw/5(Wroll), Roll Rate/1, Damp Torque Yaw1/3(w), Integrator5/1
  Integrator1/1 -> Damp Torque Yaw3/1(theta), Pitch/1
  Integrator/1 -> Yaw Rate/1, Angular Acceleration Yaw/6(Wpitch), Damp Torque Pitch/3(w), Pitc Rate/1, Integrator1/1
  Integrator3/1 -> Damp Torque Yaw2/1(theta), Yaw/1
  Damp Torque Yaw2/1(y) -> Gain2/1
  Damp Torque Yaw3/1(y) -> Gain3/1
  Gain2/1 -> Add1/3
  Gain3/1 -> Add/3
  Damp Torque Yaw4/1(y) -> Gain5/1
  Integrator5/1 -> Damp Torque Yaw4/1(theta), Roll/1
  Gain4/1 -> Add2/2
  Gain5/1 -> Add2/3

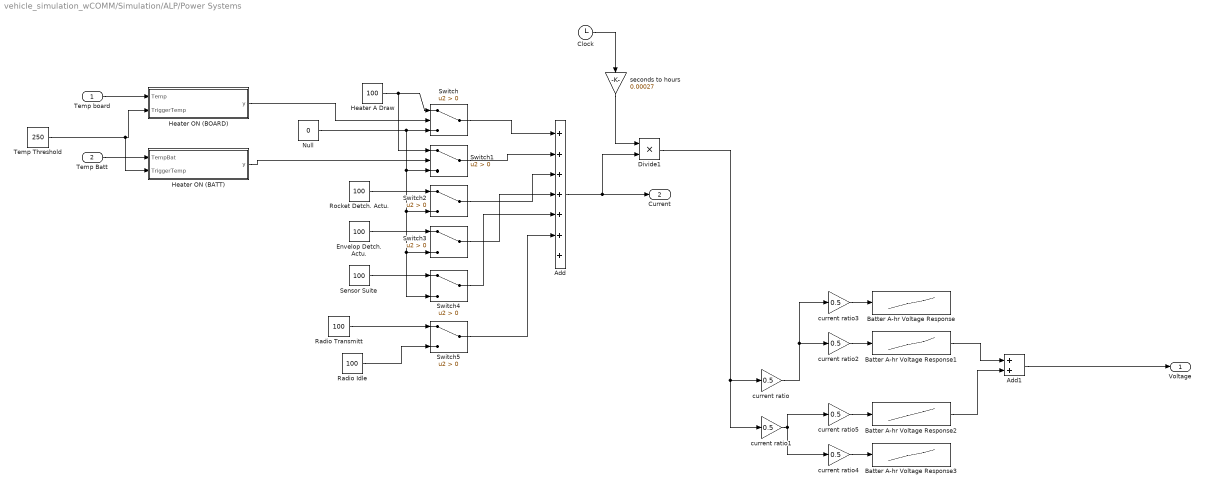
== system vehicle_simulation_wCOMM/Simulation/ALP/Power Systems ==
  Temp board : Inport
  Temp Batt : Inport  Port=2
  Add : Sum  Inputs=+++++++
  Add1 : Sum
  Batter A-hr Voltage Response{,1..3} (4 alike) : Lookup_n-D  NumberOfTableDimensions=1  BreakpointsForDimension1=[-5:5]  Table=tanh([-5:5])  InternalRulePriority=Speed  RndMeth=Simplest  InputSameDT=on
  Clock : Clock
  Divide1 : Product  Inputs=**
  Envelop Detch. Actu. : Constant  Value=100
  Heater A Draw : Constant  Value=100
  Heater ON (BATT) : MATLAB Function  TreatAsAtomicUnit=on
  Heater ON (BOARD) : MATLAB Function  TreatAsAtomicUnit=on
  Null : Constant  Value=0
  Radio Idle : Constant  Value=100
  Radio Transmitt : Constant  Value=100
  Rocket Detch. Actu. : Constant  Value=100
  Sensor Suite : Constant  Value=100
  Switch{,1..5} (6 alike) : Switch  Criteria=u2 > Threshold
  Temp Threshold : Constant  Value=250
  current ratio{,1..5} (6 alike) : Gain  Gain=0.5
  seconds to hours : Gain  Gain=0.00027
  Voltage : Outport
  Current : Outport  Port=2
  wires:
  Heater A Draw/1 -> Switch1/1, Switch/1
  Null/1 -> Switch4/3, Switch3/3, Switch2/3, Switch1/3, Switch/3
  Switch/1 -> Add/1
  Rocket Detch. Actu./1 -> Switch2/1
  Envelop Detch. Actu./1 -> Switch3/1
  Sensor Suite/1 -> Switch4/1
  Radio Transmitt/1 -> Switch5/1
  Radio Idle/1 -> Switch5/3
  Switch1/1 -> Add/2
  Switch2/1 -> Add/3
  Switch3/1 -> Add/4
  Switch4/1 -> Add/5
  Switch5/1 -> Add/6
  Add/1 -> Divide1/2, Current/1
  Clock/1 -> seconds to hours/1
  seconds to hours/1 -> Divide1/1
  Divide1/1 -> current ratio1/1, current ratio/1
  current ratio/1 -> current ratio2/1, current ratio3/1
  current ratio2/1 -> Batter A-hr Voltage Response1/1
  current ratio3/1 -> Batter A-hr Voltage Response/1
  current ratio4/1 -> Batter A-hr Voltage Response3/1
  current ratio5/1 -> Batter A-hr Voltage Response2/1
  current ratio1/1 -> current ratio5/1, current ratio4/1
  Batter A-hr Voltage Response1/1 -> Add1/1
  Batter A-hr Voltage Response2/1 -> Add1/2
  Add1/1 -> Voltage/1
  Heater ON (BATT)/1(y) -> Switch1/2
  Heater ON (BOARD)/1(y) -> Switch/2
  Temp board/1 -> Heater ON (BOARD)/1(Temp)
  Temp Batt/1 -> Heater ON (BATT)/1(TempBat)
  Temp Threshold/1 -> Heater ON (BATT)/2(TriggerTemp), Heater ON (BOARD)/2(TriggerTemp)
